simulink model "sampleModel2086"  (R2023a)
settings: Solver=VariableStepAuto  StartTime=0.0  StopTime=10.0  RelTol=1e-3
libraries: hdlsllib x2, simulink x1
settings Model: Creator=user1  LastModifiedBy=user1

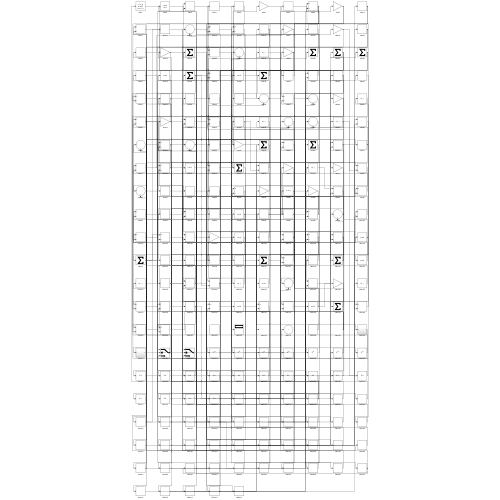
[thumbnail: Simulink's stored preview of the top-level diagram]
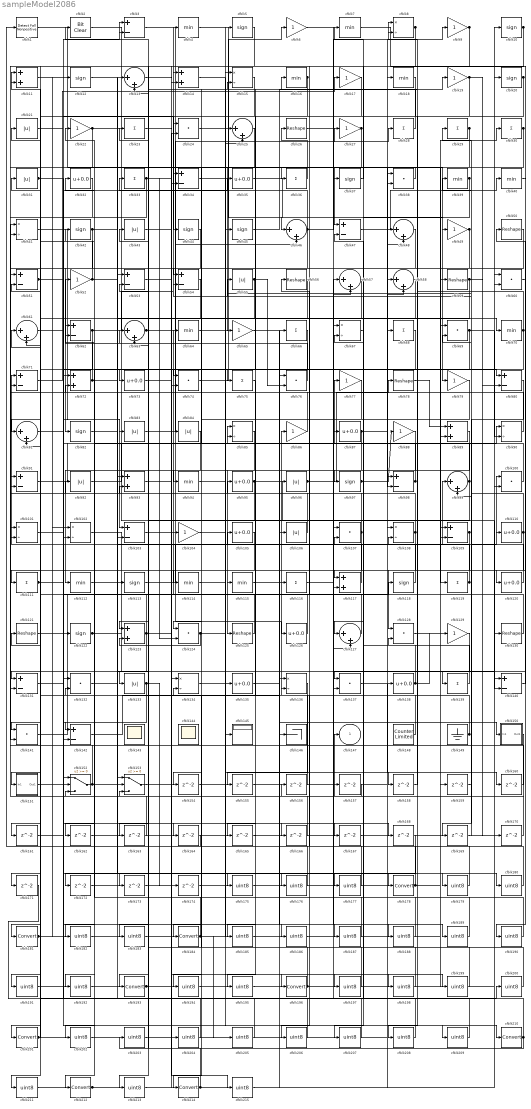
== system sampleModel2086 ==
  cfblk1 : hdlsllib/Logic and Bit Operations/Detect Fall Nonpositive  vinit=0  OutDataTypeStr=boolean
  cfblk{5,10,12,20,37,42,44..45,82,97,113,118,122} (13 alike) : Signum
  cfblk{24,38,60,69,74,76,100,107,124,128,132,137,141} (13 alike) : DotProduct  OutDataTypeStr=Inherit: Inherit via internal rule
  cfblk{8,15,41,67,85,90,101..102,108,134,136} (11 alike) : Product  Inputs=*/  RndMeth=Zero  SaturateOnIntegerOverflow=on
  cfblk{3,34,47,51,53..54,62,71,80,91,98,103,109,131,140,142} (16 alike) : Sum  Inputs=+-
  cfblk{6,9,17,19,22,27,49,52,65,77,79,86,88,104,129} (15 alike) : Gain
  cfblk{32,35,73,87,95,105,110,120,126,135,138} (11 alike) : Bias  Bias=0.0  SaturateOnIntegerOverflow=off
  cfblk{21,31,43,55,83..84,92,96,106,133} (10 alike) : Abs  SaturateOnIntegerOverflow=off
  cfblk{11,14,72,89,93,117,123} (7 alike) : Sum
  cfblk{23,28..30,33,36,66,68,75,111,116,119,139} (13 alike) : Sum  Inputs=+
  cfblk{4,7,16,18,39..40,64,70,94,112,114..115} (12 alike) : MinMax
  cfblk{26,50,56,59,78,121,125,130} (8 alike) : Reshape
  cfblk{13,25,46,48,57..58,61,63,81,99,127} (11 alike) : Sum  Inputs=|++
  cfblk143 : Scope
      settings: Floating=on
  cfblk144 : Scope
      settings: Floating=on
  cfblk145 : Display
  cfblk146 : Terminator
  cfblk148 : hdlsllib/Sources/Counter Limited  uplimit=7  tsamp=-1
  cfblk149 : Ground
  cfblk150 : Subsystem
      settings: LibrarySourceBlock=|
      | hdlsllib/Ports &
      | Subsystems/Subsystem
  cfblk151 : Subsystem
      settings: LibrarySourceBlock=|
      | hdlsllib/Ports &
      | Subsystems/Subsystem
  cfblk152 : Switch  SaturateOnIntegerOverflow=off  InputSameDT=off
  cfblk153 : Switch  SaturateOnIntegerOverflow=off  InputSameDT=off
  cfblk{154..174} (21 alike) : Delay  SampleTime=1
  cfblk{175..177,179..180,182..183,185..192,194..195,197..200,202..209,211,213,215} (32 alike) : DataTypeConversion  OutDataTypeStr=uint8  SaturateOnIntegerOverflow=off  RndMeth=Floor
  cfblk{178,181,184,193,196,201,210,212,214} (9 alike) : DataTypeConversion  SaturateOnIntegerOverflow=off  RndMeth=Floor
  cfblk2 : simulink/Logic and Bit Operations/Bit Clear  iBit=0
      settings: LibrarySourceBlock=|
      | hdlsllib/Logic and Bit
      | Operations/Bit Clear
  cfblk147 : Outport  VectorParamsAs1DForOutWhenUnconnected=off
  wires:
  cfblk49/1 -> cfblk82/1, cfblk123/1
  cfblk71/1 -> cfblk17/1
  cfblk74/1 -> cfblk29/1
  cfblk4/1 -> cfblk46/1
  cfblk41/1 -> cfblk103/1
  cfblk151/1(Out1) -> cfblk72/1
  cfblk68/1 -> cfblk214/1
  cfblk148/1 -> cfblk86/1
  cfblk3/1 -> cfblk126/1
  cfblk66/1 -> cfblk212/1
  cfblk89/1 -> cfblk125/1
  cfblk48/1 -> cfblk184/1
  cfblk78/1 -> cfblk89/1
  cfblk63/1 -> cfblk27/1, cfblk3/2
  cfblk97/1 -> cfblk88/1, cfblk117/1
  cfblk149/1 -> cfblk72/2, cfblk8/2, cfblk85/2
  cfblk11/1 -> cfblk79/1
  cfblk2/1 -> cfblk146/1
  cfblk23/1 -> cfblk196/1
  cfblk88/1 -> cfblk112/1
  cfblk83/1 -> cfblk46/2
  cfblk35/1 -> cfblk107/1
  cfblk104/1 -> cfblk210/1
  cfblk125/1 -> cfblk42/1
  cfblk46/1 -> cfblk13/2, cfblk8/1, cfblk213/1
  cfblk64/1 -> cfblk6/1
  cfblk108/1 -> cfblk128/1, cfblk96/1, cfblk117/2
  cfblk19/1 -> cfblk170/1, cfblk208/1
  cfblk7/1 -> cfblk139/1
  cfblk106/1 -> cfblk71/1
  cfblk141/1 -> cfblk64/1
  cfblk86/1 -> cfblk31/1
  cfblk26/1 -> cfblk49/1
  cfblk30/1 -> cfblk98/2, cfblk154/1
  cfblk142/1 -> cfblk116/1
  cfblk138/1 -> cfblk129/1, cfblk54/2
  cfblk55/1 -> cfblk74/1, cfblk76/2
  cfblk56/1 -> cfblk74/2
  cfblk72/1 -> cfblk52/1, cfblk140/2
  cfblk128/1 -> cfblk30/1
  cfblk29/1 -> cfblk94/1, cfblk54/1, cfblk206/1
  cfblk9/1 -> cfblk41/2, cfblk176/1
  cfblk16/1 -> cfblk81/1, cfblk153/2
  cfblk45/1 -> cfblk19/1
  cfblk122/1 -> cfblk100/1, cfblk145/1
  cfblk15/1 -> cfblk61/2
  cfblk70/1 -> cfblk16/1, cfblk172/1
  cfblk27/1 -> cfblk65/1, cfblk124/1
  cfblk18/1 -> cfblk133/1
  cfblk34/1 -> cfblk28/1
  cfblk61/1 -> cfblk122/1
  cfblk62/1 -> cfblk4/1, cfblk111/1
  cfblk14/1 -> cfblk135/1
  cfblk33/1 -> cfblk101/2, cfblk124/2, cfblk199/1
  cfblk102/1 -> cfblk105/1
  cfblk31/1 -> cfblk80/1, cfblk191/1
  cfblk1/1 -> cfblk119/1
  cfblk28/1 -> cfblk2/1
  cfblk113/1 -> cfblk108/2
  cfblk152/1 -> cfblk110/1, cfblk71/2
  cfblk96/1 -> cfblk78/1, cfblk10/1
  cfblk94/1 -> cfblk5/1
  cfblk10/1 -> cfblk63/2, cfblk177/1
  cfblk98/1 -> cfblk14/1, cfblk63/1
  cfblk47/1 -> cfblk40/1
  cfblk85/1 -> cfblk142/1
  cfblk82/1 -> cfblk113/1
  cfblk37/1 -> cfblk7/1
  cfblk119/1 -> cfblk99/1, cfblk85/1
  cfblk91/1 -> cfblk77/1
  cfblk65/1 -> cfblk150/1(In1)
  cfblk126/1 -> cfblk95/1
  cfblk112/1 -> cfblk13/1
  cfblk39/1 -> cfblk127/1, cfblk97/1
  cfblk40/1 -> cfblk120/1
  cfblk123/1 -> cfblk62/2, cfblk101/1, cfblk171/1, cfblk197/1
  cfblk5/1 -> cfblk14/2
  cfblk25/1 -> cfblk181/1
  cfblk99/1 -> cfblk15/2, cfblk185/1
  cfblk127/1 -> cfblk33/1
  cfblk87/1 -> cfblk9/1, cfblk192/1
  cfblk51/1 -> cfblk83/1, cfblk186/1
  cfblk36/1 -> cfblk26/1
  cfblk107/1 -> cfblk81/2, cfblk165/1
  cfblk20/1 -> cfblk44/1, cfblk75/1
  cfblk57/1 -> cfblk193/1
  cfblk92/1 -> cfblk59/1
  cfblk32/1 -> cfblk102/2
  cfblk12/1 -> cfblk103/2
  cfblk43/1 -> cfblk35/1
  cfblk129/1 -> cfblk137/1
  cfblk124/1 -> cfblk45/1, cfblk123/2
  cfblk110/1 -> cfblk114/1, cfblk55/1
  cfblk100/1 -> cfblk22/1
  cfblk132/1 -> cfblk178/1
  cfblk135/1 -> cfblk90/1
  cfblk121/1 -> cfblk84/1
  cfblk75/1 -> cfblk115/1
  cfblk59/1 -> cfblk131/1, cfblk80/2
  cfblk133/1 -> cfblk142/2, cfblk174/1
  cfblk44/1 -> cfblk73/1
  cfblk95/1 -> cfblk140/1, cfblk173/1
  cfblk21/1 -> cfblk24/1
  cfblk140/1 -> cfblk50/1
  cfblk109/1 -> cfblk162/1, cfblk211/1
  cfblk120/1 -> cfblk39/1
  cfblk101/1 -> cfblk3/1
  cfblk111/1 -> cfblk12/1, cfblk34/1, cfblk179/1
  cfblk22/1 -> cfblk47/1, cfblk131/2
  cfblk42/1 -> cfblk70/1, cfblk141/2
  cfblk131/1 -> cfblk118/1
  cfblk69/1 -> cfblk90/2, cfblk183/1
  cfblk50/1 -> cfblk141/1
  cfblk52/1 -> cfblk21/1, cfblk167/1
  cfblk117/1 -> cfblk91/1
  cfblk130/1 -> cfblk56/1
  cfblk139/1 -> cfblk87/1
  cfblk76/1 -> cfblk62/1
  cfblk153/1 -> cfblk147/1
  cfblk90/1 -> cfblk11/1
  cfblk8/1 -> cfblk37/1, cfblk151/1(In1), cfblk34/2
  cfblk118/1 -> cfblk91/2
  cfblk58/1 -> cfblk201/1
  cfblk17/1 -> cfblk137/2
  cfblk73/1 -> cfblk109/2
  cfblk38/1 -> cfblk36/1
  cfblk154/1 -> cfblk15/1
  cfblk79/1 -> cfblk155/1
  cfblk155/1 -> cfblk108/1
  cfblk150/1(Out1) -> cfblk156/1
  cfblk156/1 -> cfblk61/1
  cfblk157/1 -> cfblk152/3
  cfblk24/1 -> cfblk158/1
  cfblk158/1 -> cfblk128/2
  cfblk159/1 -> cfblk69/2
  cfblk137/1 -> cfblk160/1
  cfblk160/1 -> cfblk51/1
  cfblk54/1 -> cfblk161/1
  cfblk162/1 -> cfblk100/2
  cfblk84/1 -> cfblk163/1
  cfblk163/1 -> cfblk152/2
  cfblk81/1 -> cfblk164/1
  cfblk164/1 -> cfblk1/1
  cfblk103/1 -> cfblk166/1
  cfblk166/1 -> cfblk41/1
  cfblk167/1 -> cfblk38/2
  cfblk6/1 -> cfblk168/1
  cfblk80/1 -> cfblk169/1
  cfblk169/1 -> cfblk99/2
  cfblk170/1 -> cfblk47/2
  cfblk172/1 -> cfblk127/2
  cfblk173/1 -> cfblk98/1
  cfblk174/1 -> cfblk18/1
  cfblk136/1 -> cfblk175/1
  cfblk175/1 -> cfblk109/1
  cfblk176/1 -> cfblk136/1
  cfblk177/1 -> cfblk136/2
  cfblk178/1 -> cfblk157/1, cfblk92/1
  cfblk179/1 -> cfblk132/1
  cfblk114/1 -> cfblk180/1
  cfblk180/1 -> cfblk132/2
  cfblk181/1 -> cfblk159/1, cfblk51/2, cfblk102/1
  cfblk168/1 -> cfblk182/1
  cfblk182/1 -> cfblk25/1
  cfblk183/1 -> cfblk25/2
  cfblk184/1 -> cfblk32/1, cfblk205/1
  cfblk185/1 -> cfblk48/1
  cfblk186/1 -> cfblk48/2
  cfblk53/1 -> cfblk187/1
  cfblk187/1 -> cfblk43/1
  cfblk116/1 -> cfblk188/1
  cfblk188/1 -> cfblk53/1
  cfblk115/1 -> cfblk189/1
  cfblk189/1 -> cfblk53/2
  cfblk60/1 -> cfblk190/1
  cfblk190/1 -> cfblk107/2
  cfblk191/1 -> cfblk60/1
  cfblk192/1 -> cfblk60/2
  cfblk193/1 -> cfblk130/1, cfblk69/1
  cfblk77/1 -> cfblk194/1
  cfblk194/1 -> cfblk57/1
  cfblk165/1 -> cfblk195/1
  cfblk195/1 -> cfblk57/2
  cfblk196/1 -> cfblk76/1, cfblk89/2
  cfblk197/1 -> cfblk23/1
  cfblk134/1 -> cfblk198/1
  cfblk198/1 -> cfblk38/1
  cfblk199/1 -> cfblk134/1
  cfblk171/1 -> cfblk200/1
  cfblk200/1 -> cfblk134/2
  cfblk201/1 -> cfblk24/2, cfblk11/2
  cfblk105/1 -> cfblk202/1
  cfblk202/1 -> cfblk58/1
  cfblk203/1 -> cfblk58/2
  cfblk93/1 -> cfblk204/1
  cfblk204/1 -> cfblk153/1
  cfblk205/1 -> cfblk93/1
  cfblk206/1 -> cfblk93/2
  cfblk67/1 -> cfblk207/1
  cfblk207/1 -> cfblk152/1
  cfblk208/1 -> cfblk67/1
  cfblk161/1 -> cfblk209/1
  cfblk209/1 -> cfblk67/2
  cfblk210/1 -> cfblk203/1, cfblk121/1
  cfblk211/1 -> cfblk104/1
  cfblk212/1 -> cfblk138/1, cfblk106/1
  cfblk213/1 -> cfblk66/1
  cfblk214/1 -> cfblk153/3, cfblk20/1
  cfblk13/1 -> cfblk215/1
  cfblk215/1 -> cfblk68/1

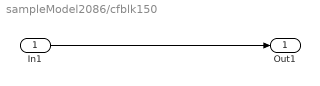
== system sampleModel2086/cfblk150 ==
  In1 : Inport
  Out1 : Outport
  wires:
  In1/1 -> Out1/1

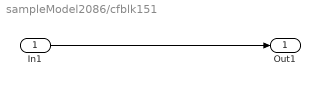
== system sampleModel2086/cfblk151 ==
  In1 : Inport
  Out1 : Outport
  wires:
  In1/1 -> Out1/1
